simulink model "REHROBLN"  (R2024a)
settings: Solver=FixedStepAuto  StartTime=0.0  StopTime=tf  FixedStep=dt  MaxStep=1e-4  RelTol=1e-5
values from neighbouring files (symbols this model uses):
  Ap = [O I; -inv(J)*C -inv(J)*B]    [RehabilitationRobotDecouplingBased_Final_version_Vlad.m]
  Bp = [O; inv(J)*Gam]    [RehabilitationRobotDecouplingBased_Final_version_Vlad.m]
  r1f = 4.0*pi/18    (= 0.698131700798)    [RehabilitationRobotDecouplingBased_Final_version_Vlad.m]
  r1i = 0    [RehabilitationRobotDecouplingBased_Final_version_Vlad.m]
  r1m = 4.5*pi/18    (= 0.785398163397)    [RehabilitationRobotDecouplingBased_Final_version_Vlad.m]
  r2f = 4.0*pi/18    (= 0.698131700798)    [RehabilitationRobotDecouplingBased_Final_version_Vlad.m]
  r2i = 0    [RehabilitationRobotDecouplingBased_Final_version_Vlad.m]
  r2m = 7.0*pi/18    (= 1.2217304764)    [RehabilitationRobotDecouplingBased_Final_version_Vlad.m]
  t1f = t1m + 2.0    (= 4.5)    [RehabilitationRobotDecouplingBased_Final_version_Vlad.m]
  t1i = 0    [RehabilitationRobotDecouplingBased_Final_version_Vlad.m]
  t1m = t1i + 2.5    (= 2.5)    [RehabilitationRobotDecouplingBased_Final_version_Vlad.m]
  t2f = t2m + 2.0    (= 4.5)    [RehabilitationRobotDecouplingBased_Final_version_Vlad.m]
  t2i = 0    [RehabilitationRobotDecouplingBased_Final_version_Vlad.m]
  t2m = t2i + 2.5    (= 2.5)    [RehabilitationRobotDecouplingBased_Final_version_Vlad.m]
undefined symbols (not defined in the file or in its folder): A4, B4, C4, D4
settings Model: Creator=KorogluH  LastModifiedBy=31629
settings SolverCC: AlgebraicLoopSolver=TrustRegion
settings DebuggingCC: UnconnectedInputMsg=warning  UnconnectedOutputMsg=warning  UnconnectedLineMsg=warning
settings ModelReferenceCC: EnableRefExpFcnMdlSchedulingChecks=on
settings SFSimCC: CustomCodeUndefinedFunction=UseInterfaceOnly
settings RTWCC: GPUComputeCapability=3.5  DLArmComputeVersion=19.05

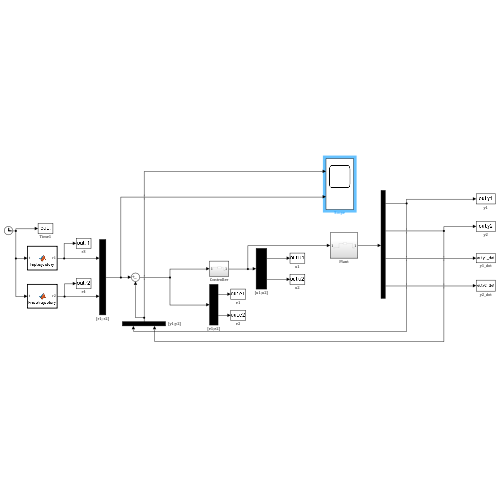
[thumbnail: Simulink's stored preview of the top-level diagram]
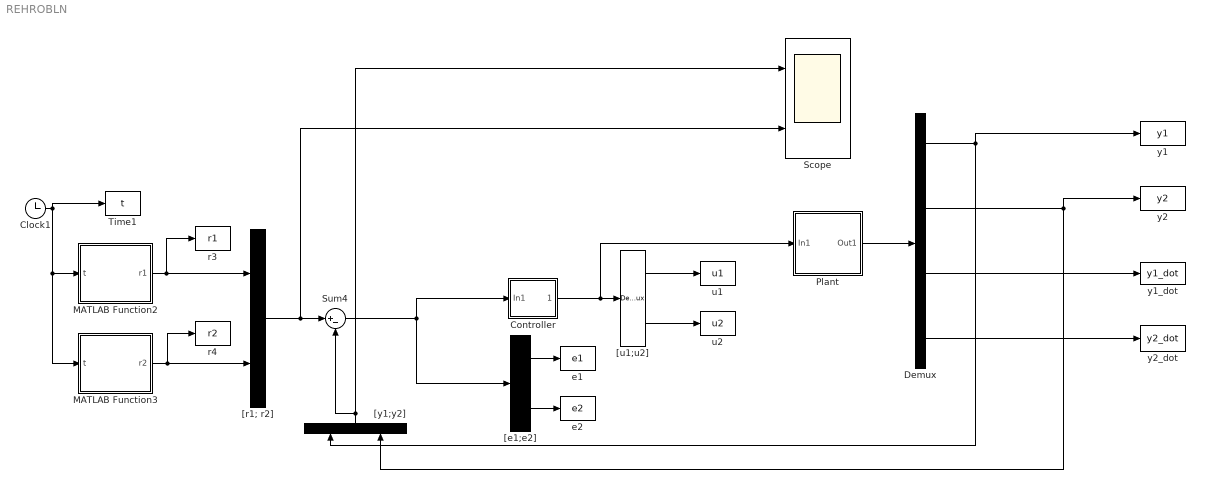
== system REHROBLN ==
  Clock1 : Clock
  Controller : Subsystem
  Demux : Demux  Outputs=[1 1 1 1]
  MATLAB Function2 : MATLAB Function  TreatAsAtomicUnit=on
  MATLAB Function3 : MATLAB Function  TreatAsAtomicUnit=on
  Plant : Subsystem
  Scope : Scope  NumInputPorts=2
  Sum4 : Sum  Inputs=|+-
  Time1 : ToWorkspace  VariableName=t  SampleTime=-1
      settings: Save2DSignal=2-D array (concatenate along first dimension)
  "[e1;e2]" : Demux  Outputs=[1 1]
  "[r1; r2]" : Mux  Inputs=[1 1]
  "[u1;u2]" : Demux  Outputs=[1 1]
  "[y1;y2]" : Mux  Inputs=[1 1]
  e1 : ToWorkspace  VariableName=e1  SampleTime=-1
  e2 : ToWorkspace  VariableName=e2  SampleTime=-1
  r3 : ToWorkspace  VariableName=r1  SampleTime=-1
  r4 : ToWorkspace  VariableName=r2  SampleTime=-1
  u1 : ToWorkspace  VariableName=u1  SampleTime=-1
      settings: Save2DSignal=2-D array (concatenate along first dimension)
  u2 : ToWorkspace  VariableName=u2  SampleTime=-1
      settings: Save2DSignal=2-D array (concatenate along first dimension)
  y1 : ToWorkspace  VariableName=y1  SampleTime=-1
      settings: Save2DSignal=2-D array (concatenate along first dimension)
  y1_dot : ToWorkspace  VariableName=y1_dot  SampleTime=-1
      settings: Save2DSignal=2-D array (concatenate along first dimension)
  y2 : ToWorkspace  VariableName=y2  SampleTime=-1
      settings: Save2DSignal=2-D array (concatenate along first dimension)
  y2_dot : ToWorkspace  VariableName=y2_dot  SampleTime=-1
      settings: Save2DSignal=2-D array (concatenate along first dimension)
  wires:
  "[r1; r2]"/1 -> Scope/2, Sum4/1
  "[u1;u2]"/2 -> u2/1
  Demux/1 -> y1/1, "[y1;y2]"/1
  Demux/2 -> y2/1, "[y1;y2]"/2
  "[u1;u2]"/1 -> u1/1
  "[y1;y2]"/1 -> Scope/1, Sum4/2
  Demux/3 -> y1_dot/1
  Demux/4 -> y2_dot/1
  "[e1;e2]"/1 -> e1/1
  "[e1;e2]"/2 -> e2/1
  MATLAB Function3/1(r2) -> "[r1; r2]"/2, r4/1
  MATLAB Function2/1(r1) -> "[r1; r2]"/1, r3/1
  Clock1/1 -> Time1/1, MATLAB Function3/1(t), MATLAB Function2/1(t)
  Controller/1(Out1) -> Plant/1(In1), "[u1;u2]"/1
  Sum4/1 -> Controller/1(In1), "[e1;e2]"/1
  Plant/1(Out1) -> Demux/1

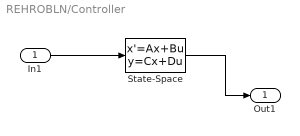
== system REHROBLN/Controller ==
  In1 : Inport
  State-Space : StateSpace  A=A4  B=B4  C=C4  D=D4  InitialCondition=0
  Out1 : Outport
  wires:
  State-Space/1 -> Out1/1
  In1/1 -> State-Space/1

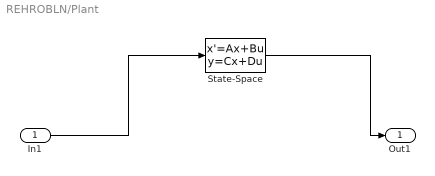
== system REHROBLN/Plant ==
  In1 : Inport
  State-Space : StateSpace  A=Ap  B=Bp  C=eye(4)  D=zeros(4,2)  InitialCondition=0
  Out1 : Outport
  wires:
  In1/1 -> State-Space/1
  State-Space/1 -> Out1/1

== matlab function REHROBLN/MATLAB Function2 ==
  data: t input; r1 output; t1i parameter; t1m parameter; t1f parameter; r1i parameter; r1m parameter; r1f parameter
function r1 = hiptrajectory(t, t1i, t1m, t1f, r1i, r1m, r1f)

if t<t1i
    r1 = r1i;
elseif t < t1m
    r1 = r1i + (r1m-r1i)*((t-t1i)/(t1m-t1i) - sin(2*pi*(t-t1i)/(t1m-t1i))/(2*pi));
elseif t < t1f
    r1 = r1m + (r1f-r1m)*((t-t1m)/(t1f-t1m) - sin(2*pi*(t-t1m)/(t1f-t1m))/(2*pi));
else
    r1 = r1f;
end

== matlab function REHROBLN/MATLAB Function3 ==
  data: t input; r2 output; t2i parameter; t2m parameter; t2f parameter; r2i parameter; r2m parameter; r2f parameter
function r2 = kneetrajectory(t, t2i, t2m, t2f, r2i, r2m, r2f)

if t<t2i
    r2 = r2i;
elseif t < t2m
    r2 = r2i + (r2m-r2i)*((t-t2i)/(t2m-t2i) - sin(2*pi*(t-t2i)/(t2m-t2i))/(2*pi));
elseif t < t2f
    r2 = r2m + (r2f-r2m)*((t-t2m)/(t2f-t2m) - sin(2*pi*(t-t2m)/(t2f-t2m))/(2*pi));
else
    r2 = r2f;
end
